simulink model "flightControlSystem"  (R2025b)
settings: Solver=ode3  StartTime=0  StopTime=TFinal  FixedStep=Ts  RelTol=1e-3  EnableMultiTasking=on
undefined symbols (not defined in the file): codertarget, Controller, DiscIntNeverNeededParam, Discrete, Estimator, g, init, orient_ref, pos_ref, Sensors, Time, Ts, var_acc_angle_N, var_bias_gyr_N, var_gyro_p_N, Vehicle
libraries: simulink x37, matrix_library x15, slpidlib x4, ctrlSharedLib x4, sharedtransform x3, visiontextngfix x3, simulink_extras x2, parrotlib x2, visionsinks x2
(part 4 of 4)

== matlab function flightControlSystem/Image Processing System/MATLAB Function12 ==
  data: RGB input; isEndLine output; circleDir output
function [isEndLine, circleDir] = detectEndLine(RGB)
%#codegen
%
% detectEndLine  Detects the end-of-path marker and estimates the bearing
%                to the red circle from the drone's current position.
%
%  Input:  RGB             - uint8 [120x160x3]
%  Output: isEndLine       - logical scalar
%                            TRUE when line terminates freely mid-frame.
%          circleAngle_deg - double, bearing to circle centre (degrees)
%                            Range: -90 to +90
%                              0   = straight ahead
%                             +90  = directly right
%                             -90  = directly left
%                            Clamped to [-90, 90]: the circle is always
%                            in the forward hemisphere by construction.
%                            Returns 0.0 when isEndLine is false.
%          circleDir       - int8 direction flag
%                             -1 = circle is to the LEFT
%                              0 = circle is straight ahead (deadband 10 deg)
%                             +1 = circle is to the RIGHT
%                            Returns int8(0) when isEndLine is false.
%
%  ANGLE CONVENTION
%  The drone camera is nadir (pointing down). In the image:
%    Row increases downward  = drone forward direction
%    Col increases rightward = drone right direction
%  Raw angle = atan2(dc_hat, dr_hat), then clamped to [-90, 90].
%  STRAIGHT_DEADBAND_DEG = 10: within +/-10 deg, circleDir = 0.
%
% ═══════════════════════════════════════════════════════════════════════════
%  PHYSICAL SETUP
% ═══════════════════════════════════════════════════════════════════════════
%
%  End marker = follow line tip + red circle (20 cm diameter) whose centre
%  is 0.3 m from the line end, on the axis of the line.
%
%  From the camera the geometry looks like one of these, depending on
%  how much of the scene is in frame:
%
%    Far view (circle visible):        Close view (circle off-screen):
%    ┌─────────────────────┐           ┌─────────────────────┐
%    │      [ circle ]     │           │    [ line ... ]     │
%    │                     │           │    [  ends   ]      │
%    │      [  line  ]     │           │    [  here  ]◄──── │
%    │      [  line  ]     │           │                     │
%    │      [  line  ]     │           │    (lots of empty)  │
%    └─────────────────────┘           └─────────────────────┘
%
%    Starting frame (this image):
%    ┌─────────────────────┐
%    │           ╱         │  ← line is diagonal, exits top edge
%    │         ╱           │  ← bottom end terminates freely mid-frame
%    │       ╱  ←end here  │
%    │                     │  ← 48+ rows of empty space below
%    └─────────────────────┘
%
% ═══════════════════════════════════════════════════════════════════════════
%  DETECTION STRATEGY
% ═══════════════════════════════════════════════════════════════════════════
%
%  Step 1 — Colour mask + opening  →  BW_all
%
%  Step 2 — Find MAIN LINE blob (corridor-based, same as detectRedLine)
%    Line criteria: area >= MIN_LINE_AREA, aspect ratio h/w >= MIN_ASPECT
%    The blob with the most pixels in the central corridor (cols 55-105)
%    is the main line.
%
%  Step 3 — Fit line axis direction
%    Compute per-row column centroid → polyfit(rows, cols, 1) → slope m.
%    The line runs in direction (dr=1, dc=m) along rows.
%
%  Step 4 — Measure FREE SPACE beyond each end along the fitted axis
%    Walk one step at a time in direction (+1, +m) from the bottom end
%    and (-1, -m) from the top end, counting steps until hitting a frame
%    edge or another red blob.
%    free_top = steps until exit/blob from top end
%    free_bot = steps until exit/blob from bottom end
%
%  Step 5 — Identify the TERMINAL end
%    terminal = whichever end has the larger free space.
%
%  Step 6 — Termination test
%    isTerminal = (terminal_free > MIN_FREE_PX)       — enough space
%              AND NOT at_frame_edge(terminal_end)    — not just exiting
%
%    "at_frame_edge" = terminal end row or column is within EDGE_MARGIN
%    pixels of any image border.  A line that continues off-frame has
%    its end within EDGE_MARGIN; a line that genuinely terminates has
%    its end in the interior.
%
%  Step 7 — Circle confirmation (bonus, not required for TRUE)
%    If ANY other red blob exists beyond the terminal end (on the far side
%    along the line axis) AND it is more compact than a line (aspect < 3),
%    set circleFound = true.  This is informational — isEndLine is already
%    set by Step 6 alone.
%
%    isEndLine = isTerminal   (circle confirmation strengthens confidence
%                              but is not gated — circle may be off-screen)
%
% ═══════════════════════════════════════════════════════════════════════════
%  CASE COVERAGE
% ═══════════════════════════════════════════════════════════════════════════
%
%  Normal following (line exits frame edge):
%    → terminal end within EDGE_MARGIN → at_frame_edge=true → FALSE  ✓
%
%  End-line approach, circle fully visible:
%    → line terminates mid-frame, circle blob found beyond it → TRUE   ✓
%
%  End-line approach, circle off-screen (starting frame):
%    → line terminates mid-frame, free_bot > MIN_FREE → TRUE           ✓
%
%  End-line approach, circle partially cut at frame edge:
%    → line terminates mid-frame → TRUE                                ✓
%    → circle blob partially visible confirms it
%
%  Normal corner turn (line bends, not a terminal):
%    → arch blob has high width ratio and std → isWidthConsistent=false → FALSE  ✓
%    → (also: both ends typically exit frame edges)
%
% ═══════════════════════════════════════════════════════════════════════════

    %% ── Startup lockout ──────────────────────────────────────────────────
    %
    %  The drone starts directly above the end marker, so the line
    %  terminates mid-frame from the very first frame.  Without a lockout
    %  the function would fire TRUE immediately on launch.
    %
    %  Strategy: count calls at the known camera frame rate (30 fps) and
    %  return FALSE for the first LOCKOUT_SECONDS regardless of what the
    %  image contains.  Uses a persistent counter so no wall-clock call
    %  is needed (compatible with Simulink codegen).
    %
    %  LOCKOUT_SECONDS = 5  →  5 × 30 = 150 frames suppressed.
    %  Adjust CAMERA_FPS if your Simulink camera block runs at a
    %  different rate.

    persistent callCount;
    if isempty(callCount)
        callCount = int32(0);
    end
    callCount = callCount + int32(1);

    CAMERA_FPS      = int32(30);
    LOCKOUT_SECONDS = int32(5);
    LOCKOUT_FRAMES  = CAMERA_FPS * LOCKOUT_SECONDS;   % = 150

    if callCount <= LOCKOUT_FRAMES
        isEndLine = false;
        circleAngle_deg = 0.0;
        circleDir = int8(0);
        return;
    end

    %% ── Tuning parameters ────────────────────────────────────────────────

    % Corridor for main-line detection (cols, 1-indexed)
    CORRIDOR_L      = int32(70);
    CORRIDOR_R      = int32(90);

    % Line shape thresholds
    MIN_LINE_AREA   = 100;   % px — reject tiny noise blobs
    MIN_LINE_ASPECT = 1.5;   % h/avg_width — line must be taller than wide
    MAX_LINE_WIDTH  = 50;    % px — reject huge merged blobs

    % Terminal-end detection
    MIN_FREE_PX       = 20;    % px along line axis beyond end = genuinely free
    EDGE_MARGIN       = 8;     % px from border = "line exits frame here"

    % Corner-arch rejection
    %  A sharp corner merges two line legs into one blob whose width grows
    %  dramatically from the apex toward the base.  A genuine terminal end
    %  is narrow and roughly constant in width.
    %
    %  WIDTH_RATIO_MAX: (far-end avg width) / (terminal-end avg width)
    %    Corner arch: far end is very wide → ratio ≈ 4-6x
    %    Terminal line: both ends similar width → ratio ≈ 1.0-1.5x
    %
    %  WIDTH_STD_MAX: std-dev of per-row widths across the whole blob
    %    Corner arch: width changes constantly → std ≈ 30-50 px
    %    Terminal line: constant width → std ≈ 2-5 px
    WIDTH_RATIO_MAX   = 2.5;   % reject if far end is >2.5x wider than near end
    WIDTH_STD_MAX     = 15.0;  % px — reject if row widths vary too much

    % Circle confirmation (optional)
    MAX_CIRCLE_ASPECT = 3.0; % blob width/height < this = compact (circle-like)
    MIN_CIRCLE_PX     = 6;   % minimum px to count as circle blob

    %% ── Normalise ────────────────────────────────────────────────────────
    RGBD = double(RGB) / 255.0;
    R    = RGBD(:,:,1);
    G    = RGBD(:,:,2);
    B    = RGBD(:,:,3);

    sceneBrightness = mean(mean(max(max(R,G),B)));

    %% ── Regime thresholds (identical to detectRedLine) ───────────────────
    if sceneBrightness < 0.05
        R_NORM_MIN = 0.45;  R_OVER_G = 2.00;  R_OVER_B = 1.50;  V_FLOOR = 0.009;
        useEdge    = false;
    elseif sceneBrightness < 0.15
        R_NORM_MIN = 0.80;  R_OVER_G = 8.00;  R_OVER_B = 8.00;  V_FLOOR = 0.20;
        useEdge    = false;
    elseif sceneBrightness < 0.50
        R_NORM_MIN = 0.55;  R_OVER_G = 1.40;  R_OVER_B = 1.40;  V_FLOOR = 0.12;
        useEdge    = false;
    elseif sceneBrightness < 0.75
        R_NORM_MIN = 0.45;  R_OVER_G = 1.40;  R_OVER_B = 1.40;  V_FLOOR = 0.12;
        useEdge    = false;
    elseif sceneBrightness < 0.95
        R_NORM_MIN = 0.342; R_OVER_G = 1.020; R_OVER_B = 1.050; V_FLOOR = 0.75;
        useEdge    = false;
    else
        R_NORM_MIN = 0.0;   R_OVER_G = 0.0;   R_OVER_B = 0.0;   V_FLOOR = 0.0;
        useEdge    = true;
    end

    %% ── Colour mask + opening ─────────────────────────────────────────────
    if ~useEdge
        V          = max(max(R,G),B);
        bright     = V >= V_FLOOR;
        safe_total = R + G + B + 1e-6;
        r_norm     = R ./ safe_total;
        r_dom_g    = R >= (R_OVER_G * G + 1e-6);
        r_dom_b    = R >= (R_OVER_B * B + 1e-6);
        raw_mask   = bright & (r_norm >= R_NORM_MIN) & r_dom_g & r_dom_b;
    else
        gray        = 0.299*R + 0.587*G + 0.114*B;
        grad_approx = abs(conv2(gray, [-1 0 1], 'same'));
        raw_mask    = grad_approx > 0.05;
    end

    se_open  = strel('disk', 2);
    raw_u32  = uint32(raw_mask);
    BW_all   = logical(imdilate(imerode(raw_u32, se_open), se_open) > uint32(0));

    %% ── Label blobs ───────────────────────────────────────────────────────
    L         = bwlabel(BW_all);
    numLabels = max(max(L));

    if numLabels == 0
        isEndLine = false;
        circleAngle_deg = 0.0;
        circleDir = int8(0);
        return;
    end

    %% ── Find main LINE blob via corridor scoring ──────────────────────────
    bestLabel   = int32(0);
    bestScore   = int32(-1);

    for k = 1:numLabels
        comp = (L == k);
        area = int32(sum(sum(comp)));
        if area < int32(MIN_LINE_AREA)
            continue;
        end

        % Rough aspect check — need row/col spans
        [rows_k, cols_k] = find(comp);
        h_k = double(max(rows_k) - min(rows_k) + 1);

        % Average per-row width
        totalW = 0.0;
        nRows  = int32(0);
        for r = int32(min(rows_k)):int32(max(rows_k))
            rp = find(comp(r,:));
            if ~isempty(rp)
                totalW = totalW + double(max(rp) - min(rp) + 1);
                nRows  = nRows + int32(1);
            end
        end
        avg_w = totalW / max(double(nRows), 1.0);

        if avg_w > MAX_LINE_WIDTH
            continue;
        end
        if (h_k / max(avg_w, 1.0)) < MIN_LINE_ASPECT
            continue;
        end

        corrScore = int32(sum(sum(L(:, CORRIDOR_L:CORRIDOR_R) == k)));
        if corrScore > bestScore
            bestScore = corrScore;
            bestLabel = int32(k);
        end
    end

    if bestLabel == int32(0)
        isEndLine = false;
        circleAngle_deg = 0.0;
        circleDir = int8(0);
        return;
    end

    lineComp = logical(L == bestLabel);

    %% ── Fit line axis direction via per-row centroids ─────────────────────
    [rows_line, ~] = find(lineComp);
    top_row = min(rows_line);
    bot_row = max(rows_line);

    % Accumulate per-row column centroid
    row_cent_col = zeros(120, 1);
    row_has_data = false(120, 1);
    for r = int32(top_row):int32(bot_row)
        rp = find(lineComp(r,:));
        if ~isempty(rp)
            row_cent_col(r) = (double(min(rp)) + double(max(rp))) / 2.0;
            row_has_data(r) = true;
        end
    end

    valid_rows = find(row_has_data);
    nValid = length(valid_rows);

    % Polyfit: col = m * row + b  (least squares)
    if nValid >= 2
        sum_r  = 0.0; sum_c  = 0.0;
        sum_rr = 0.0; sum_rc = 0.0;
        for i = 1:nValid
            rv = double(valid_rows(i));
            cv = row_cent_col(valid_rows(i));
            sum_r  = sum_r  + rv;
            sum_c  = sum_c  + cv;
            sum_rr = sum_rr + rv*rv;
            sum_rc = sum_rc + rv*cv;
        end
        n_d  = double(nValid);
        denom = n_d*sum_rr - sum_r*sum_r;
        if abs(denom) > 1e-6
            slope_m = (n_d*sum_rc - sum_r*sum_c) / denom;
        else
            slope_m = 0.0;   % perfectly horizontal
        end
    else
        slope_m = 0.0;
    end

    % End-point column centroids
    top_col = row_cent_col(top_row);
    bot_col = row_cent_col(bot_row);

    %% ── Measure free space beyond each end along the axis ─────────────────
    %
    %  Walk from the end point in the extrapolated direction.
    %  Increment row by ±1 and column by ±slope_m per step.
    %  Stop when: (a) out of bounds, or (b) hit another red pixel.
    %  Record step count = free space.

    % Beyond top: direction (dr=-1, dc=-slope_m)
    free_top = int32(0);
    r_f = double(top_row);
    c_f = double(top_col);
    for step = 1:200
        r_f = r_f - 1.0;
        c_f = c_f - slope_m;
        ri  = int32(round(r_f));
        ci  = int32(round(c_f));
        if ri < int32(1) || ri > int32(120) || ci < int32(1) || ci > int32(160)
            free_top = int32(step);
            break;
        end
        if BW_all(ri, ci) && ~lineComp(ri, ci)
            free_top = int32(step);
            break;
        end
        free_top = int32(step);
    end

    % Beyond bottom: direction (dr=+1, dc=+slope_m)
    free_bot = int32(0);
    r_f = double(bot_row);
    c_f = double(bot_col);
    for step = 1:200
        r_f = r_f + 1.0;
        c_f = c_f + slope_m;
        ri  = int32(round(r_f));
        ci  = int32(round(c_f));
        if ri < int32(1) || ri > int32(120) || ci < int32(1) || ci > int32(160)
            free_bot = int32(step);
            break;
        end
        if BW_all(ri, ci) && ~lineComp(ri, ci)
            free_bot = int32(step);
            break;
        end
        free_bot = int32(step);
    end

    %% ── Identify terminal end ─────────────────────────────────────────────
    if free_top > free_bot
        term_row  = top_row;
        term_col  = top_col;
        term_free = free_top;
    else
        term_row  = bot_row;
        term_col  = bot_col;
        term_free = free_bot;
    end

    %% ── Edge proximity check ──────────────────────────────────────────────
    %
    %  A line that is simply exiting the frame will have its terminating
    %  row/col within EDGE_MARGIN of a border.  A genuinely terminating
    %  line ends in the interior.
    at_row_edge = (term_row <= EDGE_MARGIN) || (term_row >= (120 - EDGE_MARGIN));
    at_col_edge = (term_col <= double(EDGE_MARGIN)) || (term_col >= double(160 - EDGE_MARGIN));
    at_frame_edge = at_row_edge || at_col_edge;

    %% ── Width-consistency check (corner-arch rejection) ─────────────────
    %
    %  Compute per-row widths for the whole line blob.
    %  At the terminal end (top N rows or bottom N rows, depending on which
    %  end is terminal) compare mean width against the opposite end.
    %  A corner arch has a narrow apex (terminal end) and a very wide base
    %  (far end) → ratio far/near >> 1.
    %  Additionally check the overall std-dev of widths.

    BAND_ROWS = int32(10);   % rows to average at each end for ratio check

    all_widths_vec  = zeros(120, 1);
    nWidthRows      = int32(0);
    top_band_w      = 0.0;
    top_band_n      = int32(0);
    bot_band_w      = 0.0;
    bot_band_n      = int32(0);

    for r = int32(top_row):int32(bot_row)
        rp = find(lineComp(r,:));
        if ~isempty(rp)
            rw = double(max(rp) - min(rp) + 1);
            nWidthRows = nWidthRows + int32(1);
            all_widths_vec(nWidthRows) = rw;

            if r <= int32(top_row) + BAND_ROWS - int32(1)
                top_band_w = top_band_w + rw;
                top_band_n = top_band_n + int32(1);
            end
            if r >= int32(bot_row) - BAND_ROWS + int32(1)
                bot_band_w = bot_band_w + rw;
                bot_band_n = bot_band_n + int32(1);
            end
        end
    end

    avg_top_w = top_band_w / max(double(top_band_n), 1.0);
    avg_bot_w = bot_band_w / max(double(bot_band_n), 1.0);

    % Width ratio: wide end / narrow end
    if avg_top_w > avg_bot_w
        width_ratio = avg_top_w / max(avg_bot_w, 1.0);
    else
        width_ratio = avg_bot_w / max(avg_top_w, 1.0);
    end

    % Width std-dev
    if nWidthRows > int32(1)
        w_mean = 0.0;
        for i = 1:nWidthRows
            w_mean = w_mean + all_widths_vec(i);
        end
        w_mean = w_mean / double(nWidthRows);
        w_var  = 0.0;
        for i = 1:nWidthRows
            diff_w = all_widths_vec(i) - w_mean;
            w_var  = w_var + diff_w * diff_w;
        end
        width_std = sqrt(w_var / double(nWidthRows));
    else
        width_std = 0.0;
    end

    isWidthConsistent = (width_ratio <= WIDTH_RATIO_MAX) && (width_std <= WIDTH_STD_MAX);

    %% ── Terminal-end decision ─────────────────────────────────────────────
    isTerminal = (term_free >= int32(MIN_FREE_PX)) && (~at_frame_edge) && isWidthConsistent;

    %% ── Circle confirmation (optional, strengthens confidence) ───────────
    %
    %  Look for any other blob that:
    %    - Is beyond the terminal end (dot-product check along line direction)
    %    - Has a compact shape (width/height < MAX_CIRCLE_ASPECT)
    %  Circle is NOT required — isEndLine is set by isTerminal alone.
    %  (Circle may be off-screen when drone is close to the end marker.)

    % direction unit vector from line axis
    dr_axis = 1.0;
    dc_axis = slope_m;
    axis_len = sqrt(dr_axis^2 + dc_axis^2);
    dr_hat = dr_axis / max(axis_len, 1e-6);
    dc_hat = dc_axis / max(axis_len, 1e-6);

    % If terminal is top end, flip direction (circle is "above" top end)
    if free_top > free_bot
        dr_hat = -dr_hat;
        dc_hat = -dc_hat;
    end

    circleFound = false;
    for k = 1:numLabels
        if int32(k) == bestLabel
            continue;
        end
        comp_k = (L == k);
        area_k = sum(sum(comp_k));
        if area_k < MIN_CIRCLE_PX
            continue;
        end

        [rows_k, cols_k] = find(comp_k);
        blob_row_c = (double(min(rows_k)) + double(max(rows_k))) / 2.0;
        blob_col_c = (double(min(cols_k)) + double(max(cols_k))) / 2.0;

        % Vector from terminal end to blob centre
        dr_to = blob_row_c - double(term_row);
        dc_to = blob_col_c - term_col;

        % Must be on the far side (positive projection along axis direction)
        proj = dr_to * dr_hat + dc_to * dc_hat;
        if proj < double(MIN_FREE_PX) / 2.0
            continue;
        end

        % Must be compact
        h_k = double(max(rows_k) - min(rows_k) + 1);
        w_k = double(max(cols_k) - min(cols_k) + 1);
        aspect_k = w_k / max(h_k, 1.0);
        if aspect_k < MAX_CIRCLE_ASPECT && (1.0/aspect_k) < MAX_CIRCLE_ASPECT
            circleFound = true;
            break;
        end
    end

    %% ── Final result ──────────────────────────────────────────────────────
    isEndLine = isTerminal;

    % Optional: require circle confirmation for extra robustness.
    % Uncomment the line below if false positives are a problem in flight.
    isEndLine = isTerminal && (circleFound || term_free > int32(MIN_FREE_PX * 2))

    %% ── Circle bearing angle and direction flag ──────────────────────────
    %
    %  The circle lies along the line axis beyond the terminal end.
    %  (dr_hat, dc_hat) already points in that direction.
    %
    %  Raw angle = atan2(dc_hat, dr_hat) in degrees.
    %    dc_hat encodes left/right  (+dc = right)
    %    dr_hat encodes fwd/back    (+dr = forward)
    %
    %  The circle is always in the FORWARD hemisphere (the line points
    %  toward it and the drone follows the line forward). So the raw
    %  angle from atan2 is already in [-90, 90] for the normal case.
    %  We clamp explicitly to handle floating-point edge cases.
    %
    %  circleDir flag with 10-degree deadband:
    %    angle in (-10, +10) -> 0  (straight)
    %    angle <= -10        -> -1 (left)
    %    angle >= +10        -> +1 (right)

    STRAIGHT_DEADBAND_DEG = 10.0;
    isEndLine

    if isEndLine
        raw_angle = atan2(dc_hat, dr_hat) * (180.0 / pi);

        % Clamp to [-90, 90]
        % circleAngle = mod(raw_angle,180) - 180;
        % circleAngle_deg = min(max(circleAngle,-135),135)
        circleAngle_deg = raw_angle;
        % Direction flag
        if circleAngle_deg >= STRAIGHT_DEADBAND_DEG
            circleDir = int8(1);    % right
        elseif circleAngle_deg <= -STRAIGHT_DEADBAND_DEG
            circleDir = int8(-1);   % left
        else
            circleDir = int8(0);    % straight
        end
    else
        circleAngle_deg = 0.0;
        circleDir = int8(0);
    end

end

== matlab function flightControlSystem/Image Processing System/MATLAB Function13 ==
  data: bottom input; top input; yaw_dir_fs output
function yaw_dir_fs = fcn(bottom, top)

if top > bottom
    yaw_dir_fs = -1;
elseif bottom > top
    yaw_dir_fs = 1;
else
    yaw_dir_fs = 0;
end

end
